simulink model "Trajectory_closest_point_info_get"  (R2021a)
settings: configuration reference "AION_IDS_Speedgoat" (kept outside this file)
undefined symbols (not defined in the file): CLOSEST_DISTANCE_THRESHOLD, DEG2RAD, DELTA_ANGLE_COMPENSATION1, DELTA_ANGLE_COMPENSATION2, DELTA_ANGLE_DIVISOR360, DELTA_ANGLE_THRESHOLD, N_ALTERNATIVE_CLOSEST_POINT_QUEUE, SINGLE_STEP_MOTION_ARC_LENGTH_THRESHOLD
libraries: simulink x7
(part 2 of 2)

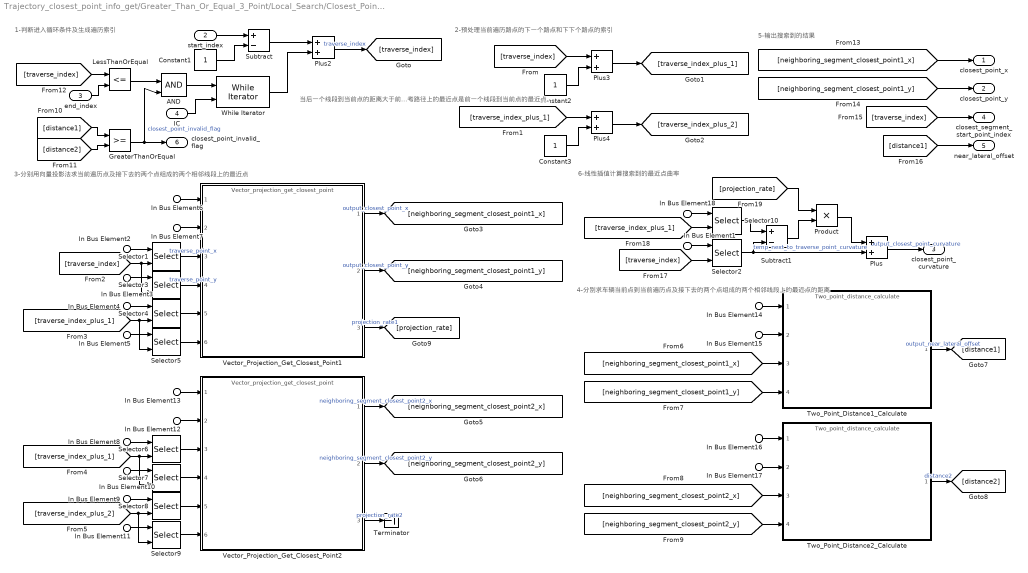
== system Trajectory_closest_point_info_get/Greater_Than_Or_Equal_3_Point/Local_Search/Closest_Point_Search_Loop ==
  note: 当后一个线段到当前点的距离大于前一个线段时，说明参考路径上的最近点是前一个线段到当前点的最近点。
  note: 6-线性插值计算搜索到的最近点曲率
  note: 5-输出搜索到的结果
  note: 4-分别求车辆当前点到当前遍历点及接下去的两个点组成的两个相邻线段上的最近点的距离
  note: 3-分别用向量投影法求当前遍历点及接下去的两个点组成的两个相邻线段上的最近点
  note: 2-预处理当前遍历路点的下一个路点和下下个路点的索引
  note: 1-判断进入循环条件及生成遍历索引
  In Bus Element{2,4,8..9} (4 alike) : Inport  PortName=input_bus  Element=trajectory_x
  In Bus Element{3,5,10..11} (4 alike) : Inport  PortName=input_bus  Element=trajectory_y
  In Bus Element{6,13..14,16} (4 alike) : Inport  PortName=input_bus  Element=current_point_x
  In Bus Element{7,12,15,17} (4 alike) : Inport  PortName=input_bus  Element=current_point_y
  In Bus Element1 : Inport  PortName=input_bus  Element=trajectory_curvature
  In Bus Element18 : Inport  PortName=input_bus  Element=trajectory_curvature
  start_index : Inport  Description=快速搜索的起始点索引，自然数，无量纲。  Port=2  OutDataTypeStr=int32  Interpolate=off
  end_index : Inport  Description=快速搜索的结束点索引，自然数，无量纲。  Port=3  OutDataTypeStr=int32  Interpolate=off
  IC : Inport  Port=4
  AND : Logic  Description=|  IconShape=distinctive  AllPortsSameDT=off  OutDataTypeStr=boolean
      | 当下列任意条件不满足时，退出循环，输出搜索到的最近点信息。
      | （1）当前遍历路点索引小于等于结束索引。
      | （2）前一个线段到当前点的距离大于等于后一个线段的。
      | 当后一个线段到当前点的距离大于前一个线段时，说明参考路径上的最近点是前一个线段到当前点的最近点。
  Constant1 : Constant  OutDataTypeStr=int32  SampleTime=-1
  Constant2 : Constant  OutDataTypeStr=int32  SampleTime=-1
  Constant3 : Constant  OutDataTypeStr=int32  SampleTime=-1
  GreaterThanOrEqual : RelationalOperator  Description=当后一个线段到当前点的距离大于前一个线段时，说明参考路径上的最近点是前一个线段到当前点的最近点，可以退出循环。  OutDataTypeStr=boolean  RndMeth=Simplest
  LessThanOrEqual : RelationalOperator  Description=当前遍历路点索引不得大于结束索引。  Operator=<=  OutDataTypeStr=boolean  RndMeth=Simplest
  Plus : Sum  Description=根据前一个线段起始点、结束点的曲率线性插值得到最近点的曲率。
  Plus2 : Sum  Description=将快速搜索起始点索引加上当前循环索引，实现顺序遍历。
  Plus3 : Sum  Description=遍历索引加1，代表当前遍历路点的下一个路点。
  Plus4 : Sum  Description=遍历索引加1以后再加1，代表当前遍历路点的下下个路点。
  Product : Product  Description=按比例计算前一个线段起始点到最近点的曲率增量。
  Selector1 : Selector  Description=获取当前遍历路点的x坐标。  IndexOptions=Index vector (port)  Indices=[1 3]  OutputSizes=1
  Selector10 : Selector  Description=获取当前遍历路点的下一个路点的曲率。  IndexOptions=Index vector (port)  Indices=[1 3]  OutputSizes=1
  Selector2 : Selector  Description=获取当前遍历路点的曲率。  IndexOptions=Index vector (port)  Indices=[1 3]  OutputSizes=1
  Selector3 : Selector  Description=获取当前遍历路点的y坐标。  IndexOptions=Index vector (port)  Indices=[1 3]  OutputSizes=1
  Selector4 : Selector  Description=获取当前遍历路点的下一个路点的x坐标。  IndexOptions=Index vector (port)  Indices=[1 3]  OutputSizes=1
  Selector5 : Selector  Description=获取当前遍历路点的下一个路点的y坐标。  IndexOptions=Index vector (port)  Indices=[1 3]  OutputSizes=1
  Selector6 : Selector  Description=获取当前遍历路点的下一个路点的x坐标。  IndexOptions=Index vector (port)  Indices=[1 3]  OutputSizes=1
  Selector7 : Selector  Description=获取当前遍历路点的下一个路点的y坐标。  IndexOptions=Index vector (port)  Indices=[1 3]  OutputSizes=1
  Selector8 : Selector  Description=获取当前遍历路点的下下个路点的x坐标。  IndexOptions=Index vector (port)  Indices=[1 3]  OutputSizes=1
  Selector9 : Selector  Description=获取当前遍历路点的下下个路点的y坐标。  IndexOptions=Index vector (port)  Indices=[1 3]  OutputSizes=1
  Subtract : Sum  Description=由于循环索引是从1开始计数，需要减去1以转换为从0开始计数的遍历索引。  Inputs=+-
  Subtract1 : Sum  Description=计算前一个线段起始点到结束点的曲率增量。  Inputs=+-
  Terminator : Terminator
  Two_Point_Distance1_Calculate : ModelReference  Description=计算车辆当前点与参考轨迹上当前遍历路点和下一个路点所组成的前一个路段的最近点的距离1。  ModelNameDialog=Two_point_distance_calculate.slx  SimulationMode=Normal  ModelReferenceVersion=4.61
  Two_Point_Distance2_Calculate : ModelReference  Description=计算车辆当前点与参考轨迹上当前遍历路点的下一个路点和下下个路点所组成的后一个路段的最近点的距离2。  ModelNameDialog=Two_point_distance_calculate.slx  SimulationMode=Normal  ModelReferenceVersion=4.61
  Vector_Projection_Get_Closest_Point1 : ModelReference  Description=向量投影法获取当前遍历路点与下一个路点之间的最近点1。  ModelNameDialog=Vector_projection_get_closest_point.slx  SimulationMode=Normal  ModelReferenceVersion=4.54
  Vector_Projection_Get_Closest_Point2 : ModelReference  Description=向量投影法获取当前遍历路点的下一个路点与下下个路点之间的最近点2。  ModelNameDialog=Vector_projection_get_closest_point.slx  SimulationMode=Normal  ModelReferenceVersion=4.54
  While Iterator : WhileIterator  MaxIters=MAX_GLOBAL_TRAJECTORY_WAY_POINT_NUMBER  ResetStates=reset  ShowIterationPort=on
  closest_point_x : Outport  Description=最近点x坐标，实数，m。  OutDataTypeStr=double
  closest_point_y : Outport  Description=最近点y坐标，实数，m。  Port=2  OutDataTypeStr=double
  closest_point_curvature : Outport  Description=最近点曲率，实数，1/m。  Port=3  OutDataTypeStr=double
  closest_segment_start_point_index : Outport  Description=最近路点线段起始点索引，自然数，无量纲。  Port=4  OutDataTypeStr=int32
  near_lateral_offset : Outport  Description=最近处横向偏差，实数，m。  Port=5  OutDataTypeStr=double
  closest_point_invalid_flag : Outport  Description=最近点有效标志。  Port=6  OutDataTypeStr=boolean
  wires:
  AND/1 -> While Iterator/1
  IC/1 -> While Iterator/2
  LessThanOrEqual/1 -> AND/1
  While Iterator/1 -> Plus2/2
  In Bus Element2/1 -> Selector1/1
  [traverse_index] -> Plus3/1
  Constant2/1 -> Plus3/2
  Plus3/1 -> [traverse_index_plus_1]
  Plus4/1 -> [traverse_index_plus_2]
  Constant3/1 -> Plus4/2
  [traverse_index_plus_1] -> Plus4/1
  [traverse_index] -> Selector1/2, Selector3/2
  In Bus Element3/1 -> Selector3/1
  Selector1/1 -> Vector_Projection_Get_Closest_Point1/3  "traverse_point_x"
  Selector3/1 -> Vector_Projection_Get_Closest_Point1/4  "traverse_point_y"
  In Bus Element5/1 -> Selector5/1
  [traverse_index_plus_1] -> Selector5/2, Selector4/2
  In Bus Element4/1 -> Selector4/1
  Selector4/1 -> Vector_Projection_Get_Closest_Point1/5
  Selector5/1 -> Vector_Projection_Get_Closest_Point1/6
  In Bus Element6/1 -> Vector_Projection_Get_Closest_Point1/1
  In Bus Element7/1 -> Vector_Projection_Get_Closest_Point1/2
  In Bus Element12/1 -> Vector_Projection_Get_Closest_Point2/2
  Selector9/1 -> Vector_Projection_Get_Closest_Point2/6
  Selector8/1 -> Vector_Projection_Get_Closest_Point2/5
  In Bus Element9/1 -> Selector8/1
  [traverse_index_plus_2] -> Selector9/2, Selector8/2
  In Bus Element11/1 -> Selector9/1
  Selector7/1 -> Vector_Projection_Get_Closest_Point2/4
  Selector6/1 -> Vector_Projection_Get_Closest_Point2/3
  In Bus Element10/1 -> Selector7/1
  [traverse_index_plus_1] -> Selector7/2, Selector6/2
  In Bus Element8/1 -> Selector6/1
  In Bus Element13/1 -> Vector_Projection_Get_Closest_Point2/1
  Vector_Projection_Get_Closest_Point1/1 -> [neighboring_segment_closest_point1_x]  "output_closest_point_x"
  Vector_Projection_Get_Closest_Point1/2 -> [neighboring_segment_closest_point1_y]  "output_closest_point_y"
  Vector_Projection_Get_Closest_Point2/1 -> [neighboring_segment_closest_point2_x]  "neighboring_segment_closest_point2_x"
  Vector_Projection_Get_Closest_Point2/2 -> [neighboring_segment_closest_point2_y]  "neighboring_segment_closest_point2_y"
  In Bus Element15/1 -> Two_Point_Distance1_Calculate/2
  In Bus Element14/1 -> Two_Point_Distance1_Calculate/1
  [neighboring_segment_closest_point1_x] -> Two_Point_Distance1_Calculate/3
  [neighboring_segment_closest_point1_y] -> Two_Point_Distance1_Calculate/4
  [neighboring_segment_closest_point2_y] -> Two_Point_Distance2_Calculate/4
  [neighboring_segment_closest_point2_x] -> Two_Point_Distance2_Calculate/3
  In Bus Element16/1 -> Two_Point_Distance2_Calculate/1
  In Bus Element17/1 -> Two_Point_Distance2_Calculate/2
  Two_Point_Distance1_Calculate/1 -> [distance1]  "output_near_lateral_offset"
  Two_Point_Distance2_Calculate/1 -> [distance2]  "distance2"
  [distance1] -> GreaterThanOrEqual/1
  [distance2] -> GreaterThanOrEqual/2
  end_index/1 -> LessThanOrEqual/2
  GreaterThanOrEqual/1 -> closest_point_invalid_flag/1, AND/2  "closest_point_invalid_flag"
  [neighboring_segment_closest_point1_y] -> closest_point_y/1
  [neighboring_segment_closest_point1_x] -> closest_point_x/1
  [distance1] -> near_lateral_offset/1
  [traverse_index] -> closest_segment_start_point_index/1
  [traverse_index] -> Selector2/2
  In Bus Element1/1 -> Selector2/1
  In Bus Element18/1 -> Selector10/1
  [traverse_index_plus_1] -> Selector10/2
  Selector10/1 -> Subtract1/1
  Selector2/1 -> Subtract1/2, Plus/2  "temp_next_to_traverse_point_curvature"
  Vector_Projection_Get_Closest_Point1/3 -> [projection_rate]  "projection_rate1"
  Vector_Projection_Get_Closest_Point2/3 -> Terminator/1  "projection_rate2"
  [projection_rate] -> Product/1
  Subtract1/1 -> Product/2
  Product/1 -> Plus/1
  Plus/1 -> closest_point_curvature/1  "output_closest_point_curvature"
  Constant1/1 -> Subtract/2
  Plus2/1 -> [traverse_index]  "traverse_index"
  start_index/1 -> Subtract/1
  Subtract/1 -> Plus2/1
  [traverse_index] -> LessThanOrEqual/1

== system Trajectory_closest_point_info_get/Greater_Than_Or_Equal_3_Point/Local_Search/End_Index_Search_Loop ==
  note: 结束索引不得超过倒数第三个点，否则凑不齐3点使用向量投影法。
  note: 将参考轨迹路点数量减去1，以便在结束索引对应的点之后仍然保有2个路点，组成3点使用向量投影法。
  note: 将上周期最近线段起始点索引加上当前循环索引，实现顺序遍历，以便搜索到本轮局部搜索的尾部结束索引。
  note: 累加路点与前一路点的 线段长度 以得到参考轨迹最近点往尾部延伸弧长。
  note: 如果累计弧长超过单周期运动距离阈值，说明搜索到了上一个周期最近点之后延伸指定距离的结束点索引。
  In Bus Element1 : Inport  PortName=input_bus  Element=trajectory_segment_length
  In Bus Element2 : Inport  PortName=input_bus  Element=closest_segment_start_point_index_previous
  In Bus Element3 : Inport  PortName=input_bus  Element=way_point_number
  IC : Inport  Port=2
  AND : Logic  Description=|  IconShape=distinctive  AllPortsSameDT=off  OutDataTypeStr=boolean
      | 当下列任意条件不满足时，退出循环，输出搜索到的局部搜索结束点索引。
      | （1）累计弧长小于单周期运动距离阈值。
      | （2）遍历索引小于倒数第二个点。
      | 结束点索引不得超过倒数第三个点，否则凑不齐3点使用向量投影法。
  Compare To Constant : simulink/Logic and Bit Operations/Compare To Constant  Description=如果累计弧长超过单周期运动距离阈值，说明搜索到了上一个周期最近点之后延伸指定距离的结束点索引。  relop=<  const=SINGLE_STEP_MOTION_ARC_LENGTH_THRESHOLD  OutDataTypeStr=boolean
  Constant1 : Constant  OutDataTypeStr=int32  SampleTime=-1
  Less Than : RelationalOperator  Description=结束索引不得超过倒数第三个点，否则凑不齐3点使用向量投影法。  Operator=<  OutDataTypeStr=boolean  RndMeth=Simplest
  Plus1 : Sum  Description=累加路点与前一路点的线段长度以得到参考轨迹最近点往尾部延伸弧长。  Inputs=|++
  Plus2 : Sum  Description=将上周期最近线段起始点索引加上当前循环索引，实现顺序遍历，以便搜索到本轮局部搜索的尾部结束索引。
  Selector2 : Selector  Description=获取参考轨迹遍历索引处的路点与前一个路点之间的线段长度。  IndexOptions=Index vector (port)  Indices=[1 3]  OutputSizes=1
  Subtract : Sum  Description=将参考轨迹路点数量减去1，以便在结束索引对应的点之后仍然保有2个路点，组成3点使用向量投影法。  Inputs=+-
  Unit Delay : UnitDelay  Description=保存本次参考轨迹最近点向尾部延伸弧长循环累加结果，用于下一次循环累加。  SampleTime=-1  StateName=tail_arc_length_previous  HasFrameUpgradeWarning=on  StateMustResolveToSignalObject=on
  While Iterator : WhileIterator  MaxIters=MAX_GLOBAL_TRAJECTORY_WAY_POINT_NUMBER  ResetStates=reset  ShowIterationPort=on
  end_index : Outport  Description=快速搜索的结束点索引（从1开始计数），自然数，无量纲。  OutDataTypeStr=int32
  wires:
  Less Than/1 -> AND/2
  Unit Delay/1 -> Plus1/2
  Plus1/1 -> Unit Delay/1, Compare To Constant/1  "tail_arc_length_current"
  Constant1/1 -> Subtract/2
  In Bus Element2/1 -> Plus2/1
  In Bus Element1/1 -> Selector2/1
  Subtract/1 -> Less Than/2
  While Iterator/1 -> Plus2/2
  In Bus Element3/1 -> Subtract/1
  Selector2/1 -> Plus1/1
  Compare To Constant/1 -> AND/1
  IC/1 -> While Iterator/2
  AND/1 -> While Iterator/1
  Plus2/1 -> Selector2/2, Less Than/1, end_index/1  "end_index"

== system Trajectory_closest_point_info_get/Greater_Than_Or_Equal_3_Point/Local_Search/Start_Index_Search_Loop ==
  note: 如果累计弧长超过单周期运动距离阈值，说明搜索到了上一个周期最近点之前延伸指定距离的起始点索引。
  note: 遍历索引不得小于2，因为首个路点没有前一个路点，其间隔距离为0，不必纳入考虑。
  note: 累加路点与前一路点的 线段长度 以得到参考轨迹最近点往头部延伸弧长。
  note: 将上周期最近线段起始点索引减去当前循环索引，实现倒序遍历，以便追溯到本轮局部搜索的头部起始索引。
  note: 将上周期最近线段起始点索引加1，因为循环索引是从1开始计数的，需要抵消它。
  In Bus Element7 : Inport  PortName=input_bus  Element=trajectory_segment_length
  In Bus Element14 : Inport  PortName=input_bus  Element=closest_segment_start_point_index_previous
  IC : Inport  Port=2
  AND : Logic  Description=|  IconShape=distinctive  AllPortsSameDT=off  OutDataTypeStr=boolean
      | 当下列任意条件不满足时，退出循环，输出搜索到的局部搜索起始点索引。
      | （1）累计弧长小于单周期运动距离阈值。
      | （2）遍历索引大于等于2。
      | 遍历索引不得小于2是因为首个路点没有前一个路点，其间隔距离为0，不必纳入考虑。
  Compare To Constant : simulink/Logic and Bit Operations/Compare To Constant  Description=如果累计弧长超过单周期运动距离阈值，说明搜索到了上一个周期最近点之前延伸指定距离的起始点索引。  relop=<  const=SINGLE_STEP_MOTION_ARC_LENGTH_THRESHOLD  OutDataTypeStr=boolean
  Compare To Constant1 : simulink/Logic and Bit Operations/Compare To Constant  Description=遍历索引不得小于2，因为首个路点没有前一个路点，其间隔距离为0，不必纳入考虑。  relop=>=  const=2  OutDataTypeStr=boolean
  Constant1 : Constant  OutDataTypeStr=int32  SampleTime=-1
  Plus : Sum  Description=将上周期最近线段起始点索引加1，因为循环索引是从1开始计数的，需要抵消它。
  Plus1 : Sum  Description=累加路点与前一路点的线段长度以得到参考轨迹最近点往头部延伸弧长。  Inputs=|++
  Selector2 : Selector  Description=获取参考轨迹遍历索引处的路点与前一个路点之间的线段长度。  IndexOptions=Index vector (port)  Indices=[1 3]  OutputSizes=1
  Subtract2 : Sum  Description=将上周期最近线段起始点索引减去当前循环索引，实现倒序遍历，以便追溯到本轮局部搜索的头部起始索引。  Inputs=+-
  Unit Delay : UnitDelay  Description=保存本次参考轨迹最近点向头部延伸弧长循环累加结果，用于下一次循环累加。  SampleTime=-1  StateName=head_arc_length_previous  HasFrameUpgradeWarning=on  StateMustResolveToSignalObject=on
  While Iterator : WhileIterator  MaxIters=MAX_GLOBAL_TRAJECTORY_WAY_POINT_NUMBER  ResetStates=reset  ShowIterationPort=on
  start_index : Outport  Description=快速搜索的起始点索引（从1开始计数），自然数，无量纲。  OutDataTypeStr=int32
  wires:
  Unit Delay/1 -> Plus1/2
  Selector2/1 -> Plus1/1
  In Bus Element14/1 -> Plus/1
  Compare To Constant/1 -> AND/1
  Compare To Constant1/1 -> AND/2
  AND/1 -> While Iterator/1
  Plus/1 -> Subtract2/1
  While Iterator/1 -> Subtract2/2
  Constant1/1 -> Plus/2
  IC/1 -> While Iterator/2
  In Bus Element7/1 -> Selector2/1
  Subtract2/1 -> start_index/1, Selector2/2, Compare To Constant1/1  "start_index"
  Plus1/1 -> Unit Delay/1, Compare To Constant/1  "head_arc_length_current"

== system Trajectory_closest_point_info_get/Greater_Than_Or_Equal_3_Point/Global_Search/Closer_Point_Queue_Search_Loop/Change_Distance_Relationship ==
  search_terminate_flag : Inport  Description=通过遍历索引与参考轨迹路点数量判断搜索结束标志，布尔量，无量纲。  OutDataTypeStr=boolean  Interpolate=off
  In Bus Element18 : Inport  Port=2  PortName=input_bus
  In Bus Element19 : Inport  Port=3  PortName=calculate_result_bus
  Action Port : ActionPort  InitializeStates=reset  PropagateVarSize=During execution  ActionPortLabel=else
  Constant1 : Constant  Value=N_ALTERNATIVE_CLOSEST_POINT_QUEUE  OutDataTypeStr=int32  SampleTime=-1
  Constant2 : Constant  Description=不满足距离关系条件时，将距离关系转移标志设置为false，等待下一个满足条件的路点。  Value=0  OutDataTypeStr=boolean  SampleTime=-1
  Data Store Read1 : DataStoreRead  DataStoreName=valid_queue_length  IndexOptions=Index vector (dialog)  Indices=1  OutputSizes=1
  Data Store Write6 : DataStoreWrite  DataStoreName=distance_relationship_transition_flag  IndexOptions=Index vector (dialog)  Indices=1  OutputSizes=1
  Global_Search_Terminate : Subsystem  Description=遍历索引到了最后，结束全局搜索，如果备选序列中还有空闲，将后一个线段的最近点采纳为备选参考路径最近点。  TreatAsAtomicUnit=on
  If : If  Description=遍历索引到了最后，结束全局搜索，如果备选序列中还有空闲，将后一个线段的最近点采纳为备选参考路径最近点。  NumInputs=2  IfExpression=u1 ~= 0 & u2 ~= 0  ShowElse=off
  Less Than : RelationalOperator  Operator=<  OutDataTypeStr=boolean  RndMeth=Simplest
  valid_queue_length : Outport  Description=备选序列有效长度，自然数，无量纲。  OutDataTypeStr=int32
  wires:
  In Bus Element19/1 -> Global_Search_Terminate/2(calculate_result_bus)
  If/1 -> Global_Search_Terminate/Action
  search_terminate_flag/1 -> If/1
  Constant2/1 -> Data Store Write6/1
  Global_Search_Terminate/1(valid_queue_length) -> valid_queue_length/1
  In Bus Element18/1 -> Global_Search_Terminate/1(input_bus)
  Data Store Read1/1 -> Less Than/1
  Constant1/1 -> Less Than/2
  Less Than/1 -> If/2

== system Trajectory_closest_point_info_get/Greater_Than_Or_Equal_3_Point/Global_Search/Closer_Point_Queue_Search_Loop/Find_A_Closer_Point ==
  In Bus Element18 : Inport  PortName=input_bus
  In Bus Element19 : Inport  Port=2  PortName=calculate_result_bus
  Action Port : ActionPort  InitializeStates=reset  PropagateVarSize=During execution  ActionPortLabel=if(u1 > u2)
  Change_Distance_Relationship : Subsystem  Description=距离关系转移标志为false，说明是首次遇到满足前后线段距离关系的点，将其采纳为备选参考路径最近点。  TreatAsAtomicUnit=on
  Constant1 : Constant  Value=N_ALTERNATIVE_CLOSEST_POINT_QUEUE  OutDataTypeStr=int32  SampleTime=-1
  Data Store Read1 : DataStoreRead  DataStoreName=valid_queue_length  IndexOptions=Index vector (dialog)  Indices=1  OutputSizes=1
  Data Store Read5 : DataStoreRead  DataStoreName=distance_relationship_transition_flag  IndexOptions=Index vector (dialog)  Indices=1  OutputSizes=1
  If : If  Description=距离关系转移标志为false且有效备选序列长度小于阈值，说明是首次遇到满足前后线段距离关系的点，且备选序列中还有空闲，将其采纳为备选参考路径最近点。  NumInputs=2  IfExpression=u1 == 0 & u2 ~= 0  ShowElse=off
  Less Than : RelationalOperator  Operator=<  OutDataTypeStr=boolean  RndMeth=Simplest
  valid_queue_length : Outport  Description=备选序列有效长度，自然数，无量纲。  OutDataTypeStr=int32
  wires:
  Data Store Read5/1 -> If/1
  If/1 -> Change_Distance_Relationship/Action
  In Bus Element19/1 -> Change_Distance_Relationship/2(calculate_result_bus)
  Change_Distance_Relationship/1(valid_queue_length) -> valid_queue_length/1
  In Bus Element18/1 -> Change_Distance_Relationship/1(input_bus)
  Data Store Read1/1 -> Less Than/1
  Constant1/1 -> Less Than/2
  Less Than/1 -> If/2

== system Trajectory_closest_point_info_get/Greater_Than_Or_Equal_3_Point/Global_Search/Specific_Closest_Point_Search_Loop/Find_A_Closer_Distance_Point ==
  traverse_index : Inport  Description=当前遍历索引，自然数，无量纲。  OutDataTypeStr=int32
  Action Port : ActionPort  InitializeStates=reset  PropagateVarSize=During execution  ActionPortLabel=if(u1 >= u2)
  Data Store Read : DataStoreRead  DataStoreName=near_lateral_offset_queue  DataStoreElements=near_lateral_offset_queue  EnableIndexing=on  NumberOfDimensions=2  IndexOptions=Index vector (port),Index vector (dialog)  Indices=1,1  OutputSizes=1,1
  Data Store Write5 : DataStoreWrite  DataStoreName=closest_distance  IndexOptions=Index vector (dialog)  Indices=1  OutputSizes=1
  closest_distance : Outport  Description=备选最近点序列中与车辆当前点之间的最近距离，正实数，m。  OutDataTypeStr=double
  closest_distance_index : Outport  Description=备选最近点序列中与车辆当前点之间的距离最近的路点索引，自然数，无量纲。  Port=2  OutDataTypeStr=int32
  wires:
  traverse_index/1 -> closest_distance_index/1, Data Store Read/1  "closest_distance_index"
  Data Store Read/1 -> Data Store Write5/1, closest_distance/1  "output_closest_distance"

== system Trajectory_closest_point_info_get/Greater_Than_Or_Equal_3_Point/Global_Search/Specific_Closest_Point_Search_Loop/Find_A_Point_Less_Than_Threshold ==
  traverse_index : Inport  Description=当前遍历索引，自然数，无量纲。  OutDataTypeStr=int32
  Action Port : ActionPort  InitializeStates=reset  PropagateVarSize=During execution  ActionPortLabel=if(u1 >= u2)
  Data Store Read1 : DataStoreRead  DataStoreName=delta_angle_queue  DataStoreElements=delta_angle_queue  EnableIndexing=on  NumberOfDimensions=2  IndexOptions=Index vector (port),Index vector (dialog)  Indices=1,1  OutputSizes=1,1
  Data Store Read2 : DataStoreRead  DataStoreName=min_delta_angle  IndexOptions=Index vector (dialog)  Indices=1  OutputSizes=1
  Find_A_Smaller_Delta_Angle_Point : Subsystem  Description=找到一个与本车横摆角偏差更小的点。  TreatAsAtomicUnit=on
  If : If  NumInputs=2  IfExpression=u1 >= u2  ShowElse=off
  min_delta_angle_index : Outport  Description=备选最近点序列中与当前车辆横摆角偏差最小的路点索引，自然数，无量纲。  OutDataTypeStr=int32
  wires:
  traverse_index/1 -> Find_A_Smaller_Delta_Angle_Point/1(traverse_index), Data Store Read1/1
  Data Store Read1/1 -> If/2
  Data Store Read2/1 -> If/1
  If/1 -> Find_A_Smaller_Delta_Angle_Point/Action
  Find_A_Smaller_Delta_Angle_Point/1(min_delta_angle_index) -> min_delta_angle_index/1

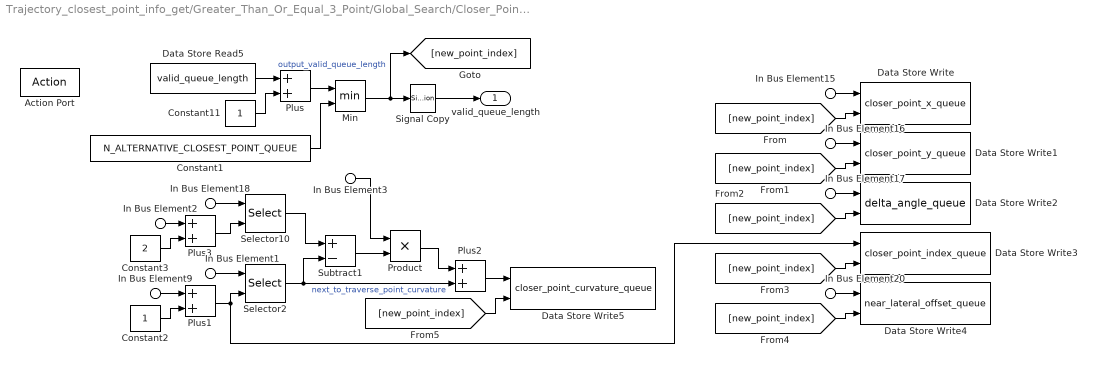
== system Trajectory_closest_point_info_get/Greater_Than_Or_Equal_3_Point/Global_Search/Closer_Point_Queue_Search_Loop/Change_Distance_Relationship/Global_Search_Terminate ==
  In Bus Element1 : Inport  PortName=input_bus  Element=trajectory_curvature
  In Bus Element18 : Inport  PortName=input_bus  Element=trajectory_curvature
  In Bus Element15 : Inport  Port=2  PortName=calculate_result_bus  Element=neighboring_segment_closest_point2_x
  In Bus Element16 : Inport  Port=2  PortName=calculate_result_bus  Element=neighboring_segment_closest_point2_y
  In Bus Element17 : Inport  Port=2  PortName=calculate_result_bus  Element=absolute_delta_angle
  In Bus Element20 : Inport  Port=2  PortName=calculate_result_bus  Element=distance2
  In Bus Element3 : Inport  Port=2  PortName=calculate_result_bus  Element=projection_rate2
  In Bus Element9 : Inport  Port=2  PortName=calculate_result_bus  Element=traverse_index
  In Bus Element2 : Inport  Port=2  PortName=calculate_result_bus  Element=traverse_index
  Action Port : ActionPort  InitializeStates=reset  PropagateVarSize=During execution  ActionPortLabel=if(u1 ~= 0 & u2 ~= 0)
  Constant1 : Constant  Value=N_ALTERNATIVE_CLOSEST_POINT_QUEUE  OutDataTypeStr=int32  SampleTime=-1
  Constant11 : Constant  OutDataTypeStr=int32  SampleTime=-1
  Constant2 : Constant  OutDataTypeStr=int32  SampleTime=-1
  Constant3 : Constant  Value=2  OutDataTypeStr=int32  SampleTime=-1
  Data Store Read5 : DataStoreRead  DataStoreName=valid_queue_length  IndexOptions=Index vector (dialog)  Indices=1  OutputSizes=1
  Data Store Write : DataStoreWrite  DataStoreName=closer_point_x_queue  DataStoreElements=closer_point_x_queue  EnableIndexing=on  NumberOfDimensions=2  IndexOptions=Index vector (port),Index vector (dialog)  Indices=1,1  OutputSizes=1,1
  Data Store Write1 : DataStoreWrite  DataStoreName=closer_point_y_queue  DataStoreElements=closer_point_y_queue  EnableIndexing=on  NumberOfDimensions=2  IndexOptions=Index vector (port),Index vector (dialog)  Indices=1,1  OutputSizes=1,1
  Data Store Write2 : DataStoreWrite  DataStoreName=delta_angle_queue  DataStoreElements=delta_angle_queue  EnableIndexing=on  NumberOfDimensions=2  IndexOptions=Index vector (port),Index vector (dialog)  Indices=1,1  OutputSizes=1,1
  Data Store Write3 : DataStoreWrite  DataStoreName=closer_point_index_queue  DataStoreElements=closer_point_index_queue  EnableIndexing=on  NumberOfDimensions=2  IndexOptions=Index vector (port),Index vector (dialog)  Indices=1,1  OutputSizes=1,1
  Data Store Write4 : DataStoreWrite  DataStoreName=near_lateral_offset_queue  DataStoreElements=near_lateral_offset_queue  EnableIndexing=on  NumberOfDimensions=2  IndexOptions=Index vector (port),Index vector (dialog)  Indices=1,1  OutputSizes=1,1
  Data Store Write5 : DataStoreWrite  DataStoreName=closer_point_curvature_queue  DataStoreElements=closer_point_curvature_queue  EnableIndexing=on  NumberOfDimensions=2  IndexOptions=Index vector (port),Index vector (dialog)  Indices=1,1  OutputSizes=1,1
  Min : MinMax  Description=最大有效备选序列长度不能超过阈值。  Inputs=2
  Plus : Sum  Description=新增一个备选点，有效备选序列长度加1。
  Plus1 : Sum  Description=计算当前遍历路点的下一个路点索引。
  Plus2 : Sum  Description=根据后一个线段起始点、结束点的曲率线性插值得到最近点的曲率。
  Plus3 : Sum  Description=计算当前遍历路点的下下个路点索引。
  Product : Product  Description=按比例计算后一个线段起始点到最近点的曲率增量。
  Selector10 : Selector  Description=获取当前遍历路点的下下个路点的曲率。  IndexOptions=Index vector (port)  Indices=[1 3]  OutputSizes=1
  Selector2 : Selector  Description=获取当前遍历路点的下一个路点的曲率。  IndexOptions=Index vector (port)  Indices=[1 3]  OutputSizes=1
  Signal Copy : SignalConversion  OverrideOpt=off
  Subtract1 : Sum  Description=计算后一个线段起始点到结束点的曲率增量。  Inputs=+-
  valid_queue_length : Outport  Description=备选序列有效长度，自然数，无量纲。  OutDataTypeStr=int32
  wires:
  Constant2/1 -> Plus1/2
  In Bus Element9/1 -> Plus1/1
  [new_point_index] -> Data Store Write2/2
  Plus/1 -> Min/1
  Constant1/1 -> Min/2
  Constant11/1 -> Plus/2
  In Bus Element17/1 -> Data Store Write2/1
  [new_point_index] -> Data Store Write1/2
  [new_point_index] -> Data Store Write3/2
  [new_point_index] -> Data Store Write4/2
  Data Store Read5/1 -> Plus/1
  Min/1 -> Signal Copy/1, [new_point_index]  "output_valid_queue_length"
  [new_point_index] -> Data Store Write/2
  In Bus Element16/1 -> Data Store Write1/1
  In Bus Element15/1 -> Data Store Write/1
  In Bus Element20/1 -> Data Store Write4/1
  In Bus Element18/1 -> Selector10/1
  Plus1/1 -> Data Store Write3/1, Selector2/2
  Product/1 -> Plus2/1
  Subtract1/1 -> Product/2
  In Bus Element1/1 -> Selector2/1
  In Bus Element3/1 -> Product/1
  Selector10/1 -> Subtract1/1
  Selector2/1 -> Subtract1/2, Plus2/2  "next_to_traverse_point_curvature"
  Plus2/1 -> Data Store Write5/1
  [new_point_index] -> Data Store Write5/2
  Constant3/1 -> Plus3/2
  In Bus Element2/1 -> Plus3/1
  Plus3/1 -> Selector10/2
  Signal Copy/1 -> valid_queue_length/1

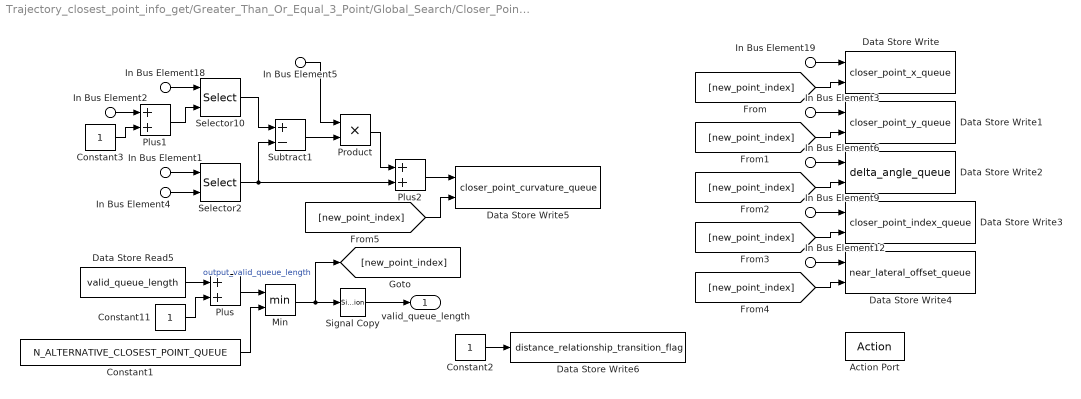
== system Trajectory_closest_point_info_get/Greater_Than_Or_Equal_3_Point/Global_Search/Closer_Point_Queue_Search_Loop/Find_A_Closer_Point/Change_Distance_Relationship ==
  In Bus Element1 : Inport  PortName=input_bus  Element=trajectory_curvature
  In Bus Element18 : Inport  PortName=input_bus  Element=trajectory_curvature
  In Bus Element19 : Inport  Port=2  PortName=calculate_result_bus  Element=neighboring_segment_closest_point1_x
  In Bus Element3 : Inport  Port=2  PortName=calculate_result_bus  Element=neighboring_segment_closest_point1_y
  In Bus Element6 : Inport  Port=2  PortName=calculate_result_bus  Element=absolute_delta_angle
  In Bus Element12 : Inport  Port=2  PortName=calculate_result_bus  Element=distance1
  In Bus Element5 : Inport  Port=2  PortName=calculate_result_bus  Element=projection_rate1
  In Bus Element9 : Inport  Port=2  PortName=calculate_result_bus  Element=traverse_index
  In Bus Element2 : Inport  Port=2  PortName=calculate_result_bus  Element=traverse_index
  In Bus Element4 : Inport  Port=2  PortName=calculate_result_bus  Element=traverse_index
  Action Port : ActionPort  InitializeStates=reset  PropagateVarSize=During execution  ActionPortLabel=if(u1 == 0 & u2 ~= 0)
  Constant1 : Constant  Value=N_ALTERNATIVE_CLOSEST_POINT_QUEUE  OutDataTypeStr=int32  SampleTime=-1
  Constant11 : Constant  OutDataTypeStr=int32  SampleTime=-1
  Constant2 : Constant  Description=修改距离关系转移标志，避免录入极近点后续的路点（因为它们都会满足距离关系条件，可却不会是最近点）。  OutDataTypeStr=boolean  SampleTime=-1
  Constant3 : Constant  OutDataTypeStr=int32  SampleTime=-1
  Data Store Read5 : DataStoreRead  DataStoreName=valid_queue_length  IndexOptions=Index vector (dialog)  Indices=1  OutputSizes=1
  Data Store Write : DataStoreWrite  DataStoreName=closer_point_x_queue  DataStoreElements=closer_point_x_queue  EnableIndexing=on  NumberOfDimensions=2  IndexOptions=Index vector (port),Index vector (dialog)  Indices=1,1  OutputSizes=1,1
  Data Store Write1 : DataStoreWrite  DataStoreName=closer_point_y_queue  DataStoreElements=closer_point_y_queue  EnableIndexing=on  NumberOfDimensions=2  IndexOptions=Index vector (port),Index vector (dialog)  Indices=1,1  OutputSizes=1,1
  Data Store Write2 : DataStoreWrite  DataStoreName=delta_angle_queue  DataStoreElements=delta_angle_queue  EnableIndexing=on  NumberOfDimensions=2  IndexOptions=Index vector (port),Index vector (dialog)  Indices=1,1  OutputSizes=1,1
  Data Store Write3 : DataStoreWrite  DataStoreName=closer_point_index_queue  DataStoreElements=closer_point_index_queue  EnableIndexing=on  NumberOfDimensions=2  IndexOptions=Index vector (port),Index vector (dialog)  Indices=1,1  OutputSizes=1,1
  Data Store Write4 : DataStoreWrite  DataStoreName=near_lateral_offset_queue  DataStoreElements=near_lateral_offset_queue  EnableIndexing=on  NumberOfDimensions=2  IndexOptions=Index vector (port),Index vector (dialog)  Indices=1,1  OutputSizes=1,1
  Data Store Write5 : DataStoreWrite  DataStoreName=closer_point_curvature_queue  DataStoreElements=closer_point_curvature_queue  EnableIndexing=on  NumberOfDimensions=2  IndexOptions=Index vector (port),Index vector (dialog)  Indices=1,1  OutputSizes=1,1
  Data Store Write6 : DataStoreWrite  DataStoreName=distance_relationship_transition_flag  IndexOptions=Index vector (dialog)  Indices=1  OutputSizes=1
  Min : MinMax  Description=最大有效备选序列长度不能超过阈值。  Inputs=2
  Plus : Sum  Description=新增一个备选点，有效备选序列长度加1。
  Plus1 : Sum  Description=计算当前遍历路点的下一个路点索引。
  Plus2 : Sum  Description=根据前一个线段起始点、结束点的曲率线性插值得到最近点的曲率。
  Product : Product  Description=按比例计算前一个线段起始点到最近点的曲率增量。
  Selector10 : Selector  Description=获取当前遍历路点的下一个路点的曲率。  IndexOptions=Index vector (port)  Indices=[1 3]  OutputSizes=1
  Selector2 : Selector  Description=获取当前遍历路点的曲率。  IndexOptions=Index vector (port)  Indices=[1 3]  OutputSizes=1
  Signal Copy : SignalConversion  OverrideOpt=off
  Subtract1 : Sum  Description=计算前一个线段起始点到结束点的曲率增量。  Inputs=+-
  valid_queue_length : Outport  Description=备选序列有效长度，自然数，无量纲。  OutDataTypeStr=int32
  wires:
  In Bus Element19/1 -> Data Store Write/1
  In Bus Element6/1 -> Data Store Write2/1
  In Bus Element9/1 -> Data Store Write3/1
  Data Store Read5/1 -> Plus/1
  Constant11/1 -> Plus/2
  Plus/1 -> Min/1
  Constant1/1 -> Min/2
  Min/1 -> [new_point_index], Signal Copy/1  "output_valid_queue_length"
  [new_point_index] -> Data Store Write/2
  In Bus Element3/1 -> Data Store Write1/1
  [new_point_index] -> Data Store Write1/2
  [new_point_index] -> Data Store Write2/2
  [new_point_index] -> Data Store Write3/2
  In Bus Element12/1 -> Data Store Write4/1
  [new_point_index] -> Data Store Write4/2
  Constant2/1 -> Data Store Write6/1
  Plus2/1 -> Data Store Write5/1
  Selector10/1 -> Subtract1/1
  Selector2/1 -> Subtract1/2, Plus2/2
  In Bus Element1/1 -> Selector2/1
  Subtract1/1 -> Product/2
  Product/1 -> Plus2/1
  In Bus Element4/1 -> Selector2/2
  In Bus Element18/1 -> Selector10/1
  [new_point_index] -> Data Store Write5/2
  In Bus Element5/1 -> Product/1
  In Bus Element2/1 -> Plus1/1
  Plus1/1 -> Selector10/2
  Constant3/1 -> Plus1/2
  Signal Copy/1 -> valid_queue_length/1

== system Trajectory_closest_point_info_get/Greater_Than_Or_Equal_3_Point/Global_Search/Specific_Closest_Point_Search_Loop/Find_A_Point_Less_Than_Threshold/Find_A_Smaller_Delta_Angle_Point ==
  traverse_index : Inport  Description=当前遍历索引，自然数，无量纲。  OutDataTypeStr=int32
  Action Port : ActionPort  InitializeStates=reset  PropagateVarSize=During execution  ActionPortLabel=if(u1 >= u2)
  Data Store Read : DataStoreRead  DataStoreName=delta_angle_queue  DataStoreElements=delta_angle_queue  EnableIndexing=on  NumberOfDimensions=2  IndexOptions=Index vector (port),Index vector (dialog)  Indices=1,1  OutputSizes=1,1
  Data Store Write5 : DataStoreWrite  DataStoreName=min_delta_angle  IndexOptions=Index vector (dialog)  Indices=1  OutputSizes=1
  min_delta_angle_index : Outport  Description=备选最近点序列中与当前车辆横摆角偏差最小的路点索引，自然数，无量纲。  OutDataTypeStr=int32
  wires:
  traverse_index/1 -> min_delta_angle_index/1, Data Store Read/1  "min_delta_angle_index"
  Data Store Read/1 -> Data Store Write5/1
